simulink model "EE_464_Sim_2"  (R2021a)
settings: Solver=VariableStepAuto  StartTime=0.0  StopTime=0.1  RelTol=1e-3
libraries: spsCurrentMeasurementLib x3, spsSeriesRLCBranchLib x2, spsRMSLib x2, spsDCVoltageSourceLib x1, spsDiodeLib x1, spsLinearTransformerLib x1, spsMosfetLib x1, spsMultimeterLib x1, spsVoltageMeasurementLib x1, spspowerguiLib x1
settings Model: Creator=EREN  LastModifiedBy=EREN

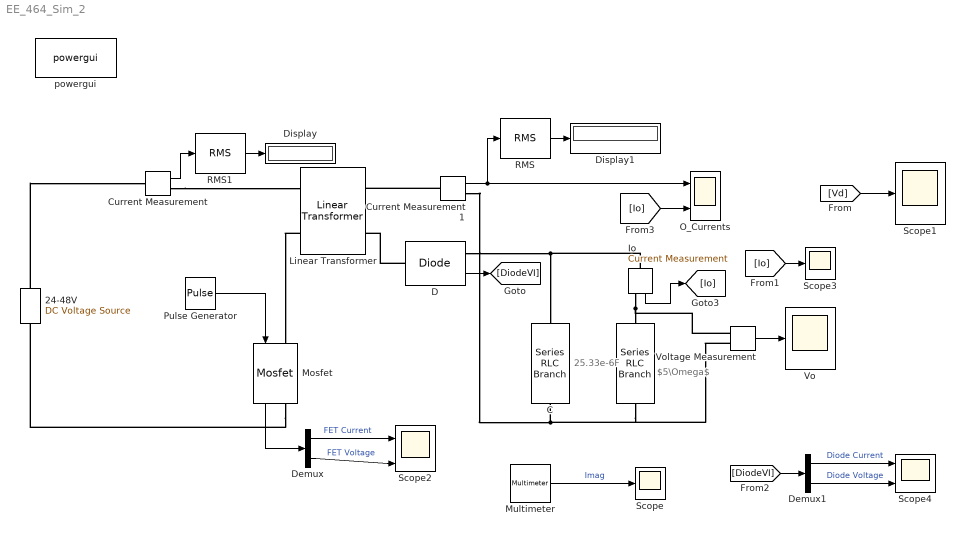
== system EE_464_Sim_2 ==
  note: 25.33e-6F
  note: $5\Omega$
  " " : spsSeriesRLCBranchLib/Series RLC Branch  LConnTagsString=__new0  RConnTagsString=__new0  BranchType=R  Resistance=5  Inductance=1e-3  SetiL0=off  InitialCurrent=0  Capacitance=1e-6  Setx0=off  InitialVoltage=0  Measurements=None
  24-48V : spsDCVoltageSourceLib/DC Voltage Source  Amplitude=48  Measurements=None
  C : spsSeriesRLCBranchLib/Series RLC Branch  LConnTagsString=__new0  RConnTagsString=__new0  BranchType=C  Resistance=1  Inductance=1e-3  SetiL0=off  InitialCurrent=0  Capacitance=25.33e-6  Setx0=off  InitialVoltage=0  Measurements=None
  Current Measurement : spsCurrentMeasurementLib/Current Measurement  PhasorSimulation=off  OutputType=Complex  PSBequivalent=0
  Current Measurement1 : spsCurrentMeasurementLib/Current Measurement  PhasorSimulation=off  OutputType=Complex  PSBequivalent=0
  D : spsDiodeLib/Diode  Ron=0.001  Lon=0  Vf=0  IC=0  UseSnubber=0  Rs=inf  Cs=0  Measurements=on
  Demux : Demux  Outputs=2
  Demux1 : Demux  Outputs=2
  Display : Display
  Display1 : Display
  Io : spsCurrentMeasurementLib/Current Measurement  PhasorSimulation=off  OutputType=Complex  PSBequivalent=0
  Linear Transformer : spsLinearTransformerLib/Linear Transformer  UNITS=SI  NominalPower=[ 45 1e5 ]  winding1=[15 0 0]  winding2=[15 0 0]  ThreeWindings=off  winding3=[3.15e+05 0.7938 0.084225]  RmLm=[inf 14.2e-6]  Measurements=Magnetization current  DataType=on
  Mosfet : spsMosfetLib/Mosfet  Ron=0  Lon=0  Rd=0  Vfd=0  IC=0  Rs=1e5  Cs=inf  Measurements=on
  Multimeter : spsMultimeterLib/Multimeter  PhasorSimulation=off  OutputType=Complex  sel=2  L=3  Gain=1  yselected={'Imag: Linear Transformer'};  PSBOutputType=1  PSBequivalent=0  AxesSetting=[0,0.1,-100,100]  Display=0  SavedBlockNames=-11
  O_Currents : Scope  NumInputPorts=2
  Pulse Generator : DiscretePulseGenerator  PulseType=Time based  Period=1/1e5  PulseWidth=23.5
  RMS : spsRMSLib/RMS  TrueRMS=on  Freq=60  RMSInit=120  Ts=0
  RMS1 : spsRMSLib/RMS  TrueRMS=on  Freq=60  RMSInit=120  Ts=0
  Scope : Scope
  Scope1 : Scope
  Scope2 : Scope  NumInputPorts=2
  Scope3 : Scope
  Scope4 : Scope  NumInputPorts=2
  Vo : Scope
  Voltage Measurement : spsVoltageMeasurementLib/Voltage Measurement  PhasorSimulation=off  OutputType=Complex  PSBequivalent=0
  powergui : spspowerguiLib/powergui  Priority=1  SimulationMode=Continuous  SampleTime=50e-6  frequency=60  Iterations=50  frequencyindice=0  Pbase=100e6  ErrMax=1e-4  UnitsV=kV  UnitsW=MW  buscounter=0  FunctionMessages=off  echomessages=off  EnableUseOfTLC=off  CurrentSourceSwitches=off  DisableSnubberDevices=off  DisableRonSwitches=off  DisableVfSwitches=off  DisplayEquations=off  AutomaticDiscreteSolvers=off  SolverType=Tustin/Backward Euler (TBE)  Interpol=off  ExternalGateDelay=off  methode=off  Ts=100  x0status=blocks  SPID=on  SwTol=0  HookPort=off  NonlinearTolerance=1e-4  nMaxIteration=100  ContinueOnMaxIteration=off  RestoreLinks=warning  ResistiveCurrentMeasurement=off  Frange=[0:2:500]  Ylog=off  Xlog=on  ShowGrid=off  save=off  variable=ZData  structure=0  ZoomFFT=off  StartTime=0.0  cycles=1  DisplayStyle=1  fundamental=60  FreqAxis=off  MaxFrequency=1000  frequencyindicesteady=1  RmsSteady=1  display=off
  wires:
  Pulse Generator/1 -> Mosfet/1
  D/1 -> [DiodeVI]
  Current Measurement1/1 -> RMS/1, O_Currents/1
  Voltage Measurement/1 -> Vo/1
  Io/1 -> [Io]
  [Io] -> O_Currents/2
  Multimeter/1 -> Scope/1  "Imag"
  Current Measurement/1 -> RMS1/1
  RMS1/1 -> Display/1
  RMS/1 -> Display1/1
  [Vd] -> Scope1/1
  Mosfet/1 -> Demux/1
  Demux/1 -> Scope2/1  "FET Current"
  Demux/2 -> Scope2/2  "FET Voltage"
  [Io] -> Scope3/1
  [DiodeVI] -> Demux1/1
  Demux1/1 -> Scope4/1  "Diode Current"
  Demux1/2 -> Scope4/2  "Diode Voltage"
  connections:
  Linear Transformer/LConn2 -- Mosfet/LConn1
  Mosfet/RConn1 -- 24-48V/LConn1
  24-48V/RConn1 -- Current Measurement/LConn1
  Current Measurement/RConn1 -- Linear Transformer/LConn1
  D/LConn1 -- Linear Transformer/RConn2
  D/RConn1 -- Io/LConn1 -- C/LConn1
  Current Measurement1/LConn1 -- Linear Transformer/RConn1
  Current Measurement1/RConn1 -- " "/RConn1 -- Voltage Measurement/LConn2 -- C/RConn1
  Io/RConn1 -- Voltage Measurement/LConn1 -- " "/LConn1
